simulink model "Serial_Send"  (R2025b)
settings: Solver=FixedStepAuto  StartTime=0.0  StopTime=100  FixedStep=0.01  RelTol=1e-3
undefined symbols (not defined in the file or in its folder): LF, u_dp_ts, u_offset
libraries: instrumentseriallib x2
settings Model: ExtModeTrigDuration=2  Creator=CoolA  LastModifiedBy=CoolA
settings SolverCC: AutoInsertRateTranBlk=on
settings OptimizationCC: EnhancedBackFolding=on  PassReuseOutputArgsAs=Individual arguments  ZeroExternalMemoryAtStartup=off  ZeroInternalMemoryAtStartup=off  MaxStackSize=64  OptimizeBlockOrder=speed  DifferentSizesBufferReuse=on  OptimizationCustomize=off  EfficientTunableParamExpr=on
settings DebuggingCC: ParameterTunabilityLossMsg=error
settings HardwareCC: ProdBitPerInt=16.0  ProdBitPerPointer=16.0  ProdBitPerSizeT=16.0  ProdBitPerPtrDiffT=16.0  ProdLargestAtomicFloat=None  ProdWordSize=8.0  ProdHWDeviceType=Atmel->AVR  UseEmbeddedCoderFeatures=off  UseSimulinkCoderFeatures=off
settings RTWCC: SystemTargetFile=ert.tlc  HardwareBoard=Arduino Uno  TemplateMakefile=ert_default_tmf  Toolchain=Arduino AVR  Description=Embedded Coder
settings CodeAppCC: ForceParamTrailComments=on  IgnoreCustomStorageClasses=off  OperatorAnnotations=on  SimulinkDataObjDesc=on  SFDataObjDesc=on  InsertBlockDesc=on
settings ERTTargetCC: ExtModeTransport=3.0  ExtModeStaticAlloc=on  ExtModeAutomaticAllocSize=off  ExtModeStaticAllocSize=250.0  ExtModeMexFile=ext_xcp  ExtModeIntrfLevel=Level2 - Open  InlinedParameterPlacement=Hierarchical  SupportContinuousTime=on  SupportNonInlinedSFcns=on  SupportVariableSizeSignals=on

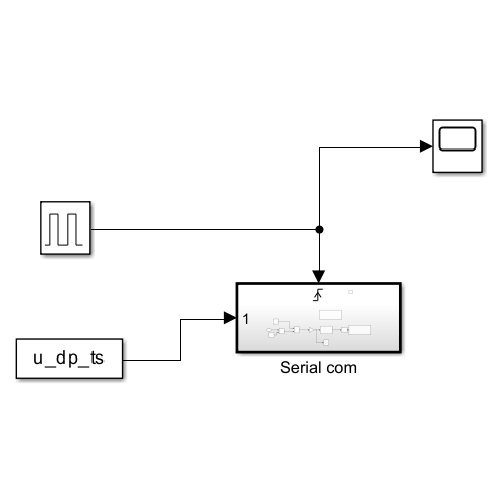
[thumbnail: Simulink's stored preview of the top-level diagram]
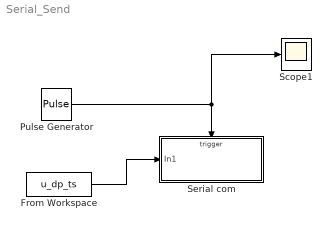
== system Serial_Send ==
  From Workspace : FromWorkspace  VariableName=u_dp_ts
  Pulse Generator : DiscretePulseGenerator  PulseType=Time based  Period=0.02  PulseWidth=50
  Scope1 : Scope
      settings: ActiveDisplayYMinimum=-1  ActiveDisplayYMaximum=1
  Serial com : Subsystem  TreatAsAtomicUnit=on
  wires:
  Pulse Generator/1 -> Serial com/Trigger, Scope1/1
  From Workspace/1 -> Serial com/1(In1)

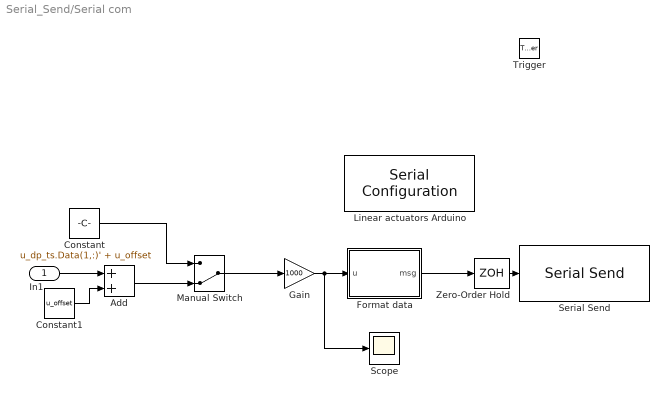
== system Serial_Send/Serial com ==
  In1 : Inport
  Trigger : TriggerPort  VariantControl=(inherit)
  Add : Sum
  Constant : Constant  Value=u_dp_ts.Data(1,:)' + u_offset
  Constant1 : Constant  Value=u_offset
  Format data : MATLAB Function  TreatAsAtomicUnit=on
  Gain : Gain  Gain=1000
  Linear actuators Arduino : instrumentseriallib/Serial Configuration  Priority=-200000  PortSel=COM7  Port=COM7  ComPort=COM7  BaudRate=115200  DataBits=8  Parity=none  StopBits=1  ByteOrder=little-endian  FlowControl=none  Timeout=10  SimulateUsing=Interpreted execution  BlockInModel=on  aMode=1
  Manual Switch : ManualSwitch  CurrentSetting=0
  Scope : Scope
      settings: ActiveDisplayYMinimum=6.8458482397932041  ActiveDisplayYMaximum=135.47435741236254
  Serial Send : instrumentseriallib/Serial Send  Priority=1  PortSel=COM7  Port=COM7  ComPort=COM7  Header=[]  Terminator=LF ('\n')  CustomTerminator=[]  EnableBlockingMode=on  SimulateUsing=Interpreted execution  BlockInModel=on  aMode=1
  Zero-Order Hold : ZeroOrderHold  SampleTime=-1
  wires:
  Zero-Order Hold/1 -> Serial Send/1
  Format data/1(msg) -> Zero-Order Hold/1
  Constant/1 -> Manual Switch/1
  Gain/1 -> Scope/1, Format data/1(u)
  Manual Switch/1 -> Gain/1
  In1/1 -> Add/1
  Add/1 -> Manual Switch/2
  Constant1/1 -> Add/2

== matlab function Serial_Send/Serial com/Format data ==
  data: u input; msg output uint8 size=[1 29]
% function msg = fcn(u)
% MAX_LEN = 30;
% u = int8(u);
% msg = sprintf('<%03d,%03d,%03d,%03d,%03d,%03d,%03d>\n', u(1), u(2), u(3), u(4), u(5), u(6), u(7));
% 
% % 03 ensures 3 digits

function msg = formatData(u)
%#codegen

MAX_LEN = 29;
msg = uint8(zeros(1, MAX_LEN));

u = int16(u);

str = sprintf('<%03d,%03d,%03d,%03d,%03d,%03d,%03d>', ...
    u(1), u(2), u(3), u(4), u(5), u(6), u(7));

len = min(length(str), MAX_LEN);
msg(1:len) = uint8(str(1:len));
